simulink model "ame532Project1_Gimbal_Tracking_R2022aVersion"  (R2023a)
settings: Solver=ode4  StartTime=0.0  StopTime=60  FixedStep=0.01  RelTol=1e-3
model workspace (MAT data in the model file):
  theta : Simulink.Parameter (value not decoded)
values from neighbouring files (symbols this model uses):
  AR_s2 = b_s2/c_s2    [computeSurfacePos.m]
  AR_s3 = b_s3/c_s3    [computeSurfacePos.m]
  AR_s4 = b_s4/c_s4    [computeSurfacePos.m]
  AR_s5 = b_s5/c_s5    [computeSurfacePos.m]
  area_s2 = c_s2 * b_s2    [computeSurfacePos.m]
  area_s3 = c_s3 * b_s3    [computeSurfacePos.m]
  area_s4 = c_s4 * b_s4    [computeSurfacePos.m]
  area_s5 = c_s5 * b_s5    [computeSurfacePos.m]
  c_s2 = componentMassesAndGeom(3,2)    [computeSurfacePos.m]
  c_s3 = componentMassesAndGeom(4,2)    [computeSurfacePos.m]
  c_s4 = componentMassesAndGeom(1,2)    [computeSurfacePos.m]
  c_s5 = componentMassesAndGeom(2,2)    [computeSurfacePos.m]
undefined symbols (not defined in the file or in its folder): a0_s2, a0_s3, a0_s4, a0_s5, CD0_s2, CD0_s3, CD0_s4, CD0_s5, CDa_s2, CDa_s3, CDa_s4, CDa_s5, CL0_s2, CL0_s3, CL0_s4, CL0_s5, CM0_s2, CM0_s3, CM0_s4, CM0_s5, CMa_s2, CMa_s3, CMa_s4, CMa_s5, e_s2, e_s3, e_s4, e_s5, earthRadius, i_s2, i_s3, i_s4, i_s5, Jxx, Jxy, Jxz, Jyx, Jyy, Jyz, Jzx, Jzy, Jzz, LL, MM, n_s2, n_s3, n_s4, n_s5, NN, rEarth, ro, x_S2_B_B, x_S3_B_B, x_S4_B_B, x_S5_B_B
libraries: simulink_extras x34, matrix_library x19, aerolibutil x7, aerolibfltsims x4, vrlib x3, aerolibtransform2 x2, sharedutil x1, simulink x1
(part 4 of 4)

== matlab function ame532Project1_Gimbal_Tracking_R2022aVersion/IMU  Aircraft dynamic sim1/aeroforce coefficient block/calculatie alpha ==
  data: i0 input; alpha output; v_B input; n_vector input; wind_w input; v_B_BA output; C_BN input
function [alpha,v_B_BA] = fcn(i0,v_B,n_vector,wind_w,C_BN)

alpha = zeros(4,1);
% this function calculates alpha that the aero surface sees

v_B_BA = v_B - C_BN*wind_w;

for i = 1:4
    alpha(i) = i0(i) - asin(dot(v_B_BA,n_vector(:,i))/norm(v_B_BA));
end

== matlab function ame532Project1_Gimbal_Tracking_R2022aVersion/IMU  Aircraft dynamic sim1/aeroforce coefficient block/extract matrix function ==
  data: aero_surface_matrix input; AR_matrix output
function AR_matrix = Extract_AR(aero_surface_matrix)

AR_matrix = aero_surface_matrix(:,7);
end

== matlab function ame532Project1_Gimbal_Tracking_R2022aVersion/IMU  Aircraft dynamic sim1/aeroforce coefficient block/extract matrix function1 ==
  data: aero_surface_matrix input; AR_matrix output
function AR_matrix = Extract_AR(aero_surface_matrix)

AR_matrix = aero_surface_matrix(:,7);
end

== matlab function ame532Project1_Gimbal_Tracking_R2022aVersion/IMU  Aircraft dynamic sim1/mass & aero property calculation/CG calculation ==
  data: M_matrix input; cg_x output; cg_y output; cg_z output
function [cg_x, cg_y, cg_z] = CG_calc(M_matrix)

mass_col = M_matrix(:,1);
x_col = M_matrix(:,5);
y_col = M_matrix(:,6);
z_col = M_matrix(:,7);

cg_x = sum(mass_col.*x_col)/(sum(mass_col));
cg_y = sum(mass_col.*y_col)/(sum(mass_col));
cg_z = sum(mass_col.*z_col)/(sum(mass_col));

end

== matlab function ame532Project1_Gimbal_Tracking_R2022aVersion/IMU  Aircraft dynamic sim1/mass & aero property calculation/MATLAB Function ==
  data: cg_location input; M_matrix input; J_matrix output
function J_matrix = fcn(cg_location,M_matrix)


mass_col = M_matrix(:,1);
x_dim = M_matrix(:,2);
y_dim = M_matrix(:,3);
z_dim = M_matrix(:,4);
x_loc = M_matrix(:,5);
y_loc = M_matrix(:,6);
z_loc = M_matrix(:,7);

Ixx = zeros(11,1);
Iyy = zeros(11,1);
Izz = zeros(11,1);
Ixz = zeros(11,1);
Izx = Ixz;
Ixy = zeros(11,1);
Iyx = Ixy;
Iyz = zeros(11,1);
Izy = Iyz;

J_matrix = zeros(3,3);

% all moment of inertial is calculated wrt to CG

for i = 1:11
    Ixx(i) = mass_col(i)*(y_dim(i)^2+z_dim(i)^2)/(12)+mass_col(i)*((y_loc(i)-cg_location(2))^2+(z_loc(i)-cg_location(3))^2); % check discussion post
    Iyy(i) = mass_col(i)*(x_dim(i)^2+z_dim(i)^2)/(12)+mass_col(i)*((x_loc(i)-cg_location(1))^2+(z_loc(i)-cg_location(3))^2);
    Izz(i) = mass_col(i)*(y_dim(i)^2+x_dim(i)^2)/(12)+mass_col(i)*((y_loc(i)-cg_location(2))^2+(x_loc(i)-cg_location(1))^2);
    Ixz(i) = mass_col(i)*((z_loc(i)-cg_location(3))*(x_loc(i)-cg_location(1)));
    Ixy(i) = mass_col(i)*((x_loc(i)-cg_location(1))*(y_loc(i)-cg_location(2)));
    Iyz(i) = mass_col(i)*((y_loc(i)-cg_location(2))*(z_loc(i)-cg_location(3)));


end

J_matrix(1,1) = sum(Ixx);
J_matrix(2,2) = sum(Iyy);
J_matrix(3,3) = sum(Izz);
J_matrix(1,2) = sum(Ixy);
J_matrix(2,1) = sum(Ixy);
J_matrix(1,3) = sum(Ixz);
J_matrix(3,1) = sum(Ixz);
J_matrix(2,3) = sum(Iyz);
J_matrix(3,2) = sum(Iyz);

J_matrix = J_matrix./1000;
end

== matlab function ame532Project1_Gimbal_Tracking_R2022aVersion/IMU  Aircraft dynamic sim1/mass & aero property calculation/MATLAB Function1 ==
  data: aero_prop_matrix input; m_matrix input; x_b_s_ac output; cg_location input
function x_b_s_ac = calculate_x_b_sb(aero_prop_matrix,m_matrix,cg_location)
%this function calculates vector of each component to CM of aircraft

x_b_sb = zeros(3,4);
x_b_s_ac = zeros(3,4);
for i = 1:4
    x_b_s_ac(:,i) = m_matrix(i,5:7)' + [0.25*aero_prop_matrix(i,4) 0 0]';
    x_b_s_ac(:,i) = x_b_s_ac(:,i)- cg_location;

%     x_b_sb(:,i) = m_matrix(i,5:7)' - cg_location;

end

== matlab function ame532Project1_Gimbal_Tracking_R2022aVersion/Gimbal Aircraft dynamic sim/Rotational Kinematics/MATLAB Function2 ==
  data: phi input; H_matrix_inv output; theta input; psi input
function H_matrix_inv = inv_h_matrix_from_euler(phi,theta,psi)

H_matrix_inv = [1, tan(theta)*sin(phi), tan(theta)*cos(phi);
                0,      cos(phi),           -sin(phi);      
                0,     sin(phi)/cos(theta),   cos(phi)/cos(theta)];

end

== matlab function ame532Project1_Gimbal_Tracking_R2022aVersion/IMU  Aircraft dynamic sim1/mass & aero property calculation/MATLAB Function2 ==
  data: M_matrix input; aero_prop output
function aero_prop = fcn(M_matrix)

aero_prop = zeros(4,7);
for i = 1:4
    aero_prop(i,1:3) = M_matrix(i,5:7);
    aero_prop(i,4) = M_matrix(i,2);
end

%% define span for each surface

    aero_prop(1,5) = M_matrix(1,3); %right wing
    aero_prop(2,5) = M_matrix(2,3); %left wing
    aero_prop(3,5) = M_matrix(3,3); %hor stab.
    aero_prop(4,5) = M_matrix(4,4); %ver stab.
%% define area and aspect ratio for each surface

for i = 1:4
    aero_prop(i,6) = aero_prop(i,4)*aero_prop(i,5);
    aero_prop(i,7) = aero_prop(i,5)/aero_prop(i,4);
end

== matlab function ame532Project1_Gimbal_Tracking_R2022aVersion/IMU  Aircraft dynamic sim1/measurement subsystem/MATLAB Function ==
  data: velocity input; magnitude output
function magnitude = magnitude_from_vector(velocity)

magnitude = sqrt(velocity(1)^2+velocity(2)^2+velocity(3)^2);

end

== matlab function ame532Project1_Gimbal_Tracking_R2022aVersion/IMU  Aircraft dynamic sim1/translational dynamics/MATLAB Function10 ==
  data: p input; Cross_Product_Matrix output; q input; r input
function Cross_Product_Matrix = omega_to_cross_product_matrix(p,q,r)

    Cross_Product_Matrix =[0 -r q; r 0 -p; -q p 0];

end

== matlab function ame532Project1_Gimbal_Tracking_R2022aVersion/Gimbal system/magnitude ==
  data: x_E_BG input; R output
function R = fcn(x_E_BG)

R = sqrt(x_E_BG(1)^2+x_E_BG(2)^2+x_E_BG(3)^2);

== matlab function ame532Project1_Gimbal_Tracking_R2022aVersion/JeoIMUmodel/Aero Forces and Moments/F&M Horiz Stab Surface (S2)/Compute Aero Lift and Drag ==
  data: v_B_E_B input; alphaLocal output; v_B_A_B input; liftSurf output; dragSurf output; AR_s2 input; i_s2 input; n_s2 input; CL0_s2 input; CD0_s2 input; CDa_s2 input; a0_s2 input; e_s2 input; ro input; area_s2 input
function [alphaLocal, liftSurf, dragSurf] = fcn(v_B_E_B, v_B_A_B, AR_s2, i_s2, n_s2, CL0_s2, CD0_s2, CDa_s2, a0_s2, e_s2, ro, area_s2)
% Compute the lift and drag forces at the respective surface
% arSurf -> Aspect Ratio of respective surfaace
% ro -> air density (note: varies with altitude)
% v_infSurf -> total airspeed at the surface, i.e. Velocity of body w.r.t Inertial/ECEF as
% measured in body frame (|V_B_E_B|)
% v_B_A_B -> relative airspeed, where it is typically 
% v_B_E_B - c_B_N * v_A_N_N and v_A_N_N is the velocity of air mass w.r.t. NED 
% nSurf_B -> Normal force applied at surface
% eSurf -> Oswald efficiency
% alphaLocal0 -> Minimum drag Angle of Attack

v_infSurf = norm(v_B_E_B);
cSurfLocAlpha = 2*pi * (AR_s2/(2+AR_s2)); % Lift coefficient at the respective surface due to the local alpha (Angle of Attack)
alphaLocal = i_s2 - asin(dot(v_B_A_B,n_s2)/norm(v_B_A_B)); % in Radians
cSurfLift = CL0_s2 + cSurfLocAlpha * alphaLocal; % Lift coefficient of surface
cSurfDrag = CD0_s2 + CDa_s2 *(alphaLocal - a0_s2)^2 + (cSurfLift^2/(pi*e_s2*AR_s2));

liftSurf = cSurfLift * 0.5 * ro * (v_infSurf^2)*area_s2;
dragSurf = cSurfDrag * 0.5 * ro * (v_infSurf^2)*area_s2;

== matlab function ame532Project1_Gimbal_Tracking_R2022aVersion/JeoIMUmodel/Aero Forces and Moments/F&M Horiz Stab Surface (S2)/Compute Aero Moment ==
  data: v_B_E_B input; momSurf output; alphaLocal input; CM0_s2 input; CMa_s2 input; ro input; area_s2 input; c_s2 input
function momSurf = fcn(v_B_E_B, alphaLocal, CM0_s2, CMa_s2, ro, area_s2, c_s2)
% Compute the Moment at the respective Surface
% v_infSurf -> total airspeed at the surface, i.e. Velocity of body w.r.t Inertial/ECEF as
% measured in body frame (|V_B_E_B|)
% ro -> air density (note: varies with altitude)
% chordSurf -> Chord of the surface area
% cSurfM0 -> Initial moment coefficient of surface
% cSurfMalpha -> Moment coefficient at the respective surface due to the
% local alpha (Angle of Attack)
v_infSurf = norm(v_B_E_B);
cSurfMom = CM0_s2 + CMa_s2*alphaLocal; % Moment coefficient of surface
momSurf = cSurfMom * 0.5 * ro * (v_infSurf^2)*area_s2 * c_s2;

== matlab function ame532Project1_Gimbal_Tracking_R2022aVersion/JeoIMUmodel/Aero Forces and Moments/F&M Horiz Stab Surface (S2)/F&M in Body/Force Due to Lift and Drag ==
  data: lift input; forceLiftDragS2_B output; drag input; v_B_E_B input; n_s2 input
function forceLiftDragS2_B = fcn(lift, drag, v_B_E_B, n_s2)

forceLiftDrag_w = lift*n_s2 - [drag; 0; 0];
alpha = atan2(v_B_E_B(3), v_B_E_B(1));
beta = asin(v_B_E_B(2) / norm(v_B_E_B));

c_S_B = [cos(alpha), 0, sin(alpha); 0, 1, 0; -sin(alpha), 0, cos(alpha)] ;
c_W_S = [cos(beta), sin(beta), 0; -sin(beta), cos(beta), 0; 0,0,1];
c_W_B = c_W_S * c_S_B;

forceLiftDragS2_B = c_W_B' * forceLiftDrag_w;

== matlab function ame532Project1_Gimbal_Tracking_R2022aVersion/JeoIMUmodel/Aero Forces and Moments/F&M Horiz Stab Surface (S2)/F&M in Body/Moment S2 ==
  data: momSurf input; momS2_B output; FliftdragS input; n_s2 input; x_S2_B_B input
function momS2_B = fcn(momSurf, FliftdragS, n_s2, x_S2_B_B)
% Compute the moment at the respective surface
crot = [0,0,0; 0,0,-1; 0,1,0];

momS2_B = momSurf * crot* n_s2 + (cross(x_S2_B_B, FliftdragS));

== matlab function ame532Project1_Gimbal_Tracking_R2022aVersion/JeoIMUmodel/Aero Forces and Moments/F&M Horiz Stab Surface (S3)/Compute Aero Lift and Drag ==
  data: v_B_E_B input; alphaLocal output; v_B_A_B input; liftSurf output; dragSurf output; AR_s3 input; i_s3 input; n_s3 input; CL0_s3 input; CD0_s3 input; CDa_s3 input; a0_s3 input; e_s3 input; ro input; area_s3 input
function [alphaLocal, liftSurf, dragSurf] = fcn(v_B_E_B, v_B_A_B, AR_s3, i_s3, n_s3, CL0_s3, CD0_s3, CDa_s3, a0_s3, e_s3, ro, area_s3)
% Compute the lift and drag forces at the respective surface
% arSurf -> Aspect Ratio of respective surfaace
% ro -> air density (note: varies with altitude)
% v_infSurf -> total airspeed at the surface, i.e. Velocity of body w.r.t Inertial/ECEF as
% measured in body frame (|V_B_E_B|)
% v_B_A_B -> relative airspeed, where it is typically 
% v_B_E_B - c_B_N * v_A_N_N and v_A_N_N is the velocity of air mass w.r.t. NED 
% nSurf_B -> Normal force applied at surface
% eSurf -> Oswald efficiency
% alphaLocal0 -> Minimum drag Angle of Attack

v_infSurf = norm(v_B_E_B);
cSurfLocAlpha = 2*pi * (AR_s3/(2+AR_s3)); % Lift coefficient at the respective surface due to the local alpha (Angle of Attack)
alphaLocal = i_s3 - asin(dot(v_B_A_B,n_s3)/norm(v_B_A_B)); % in Radians
cSurfLift = CL0_s3 + cSurfLocAlpha * alphaLocal; % Lift coefficient of surface
cSurfDrag = CD0_s3 + CDa_s3 *(alphaLocal - a0_s3)^2 + (cSurfLift^2/(pi*e_s3*AR_s3));

liftSurf = cSurfLift * 0.5 * ro * (v_infSurf^2)*area_s3;
dragSurf = cSurfDrag * 0.5 * ro * (v_infSurf^2)*area_s3;

== matlab function ame532Project1_Gimbal_Tracking_R2022aVersion/Gimbal Aircraft dynamic sim/Rotational Kinematics/MATLAB Function3 ==
  data: p input; Cross_Product_Matrix output; q input; r input
function Cross_Product_Matrix = omega_to_cross_product_matrix(p,q,r)

    Cross_Product_Matrix =[0 -r q; r 0 -p; -q p 0];

end

== matlab function ame532Project1_Gimbal_Tracking_R2022aVersion/JeoIMUmodel/Aero Forces and Moments/F&M Horiz Stab Surface (S3)/Compute Aero Moment ==
  data: v_B_E_B input; momSurf output; alphaLocal input; CM0_s3 input; CMa_s3 input; ro input; area_s3 input; c_s3 input
function momSurf = fcn(v_B_E_B, alphaLocal, CM0_s3, CMa_s3, ro, area_s3, c_s3)
% Compute the Moment at the respective Surface
% v_infSurf -> total airspeed at the surface, i.e. Velocity of body w.r.t Inertial/ECEF as
% measured in body frame (|V_B_E_B|)
% ro -> air density (note: varies with altitude)
% chordSurf -> Chord of the surface area
% cSurfM0 -> Initial moment coefficient of surface
% cSurfMalpha -> Moment coefficient at the respective surface due to the
% local alpha (Angle of Attack)
v_infSurf = norm(v_B_E_B);
cSurfMom = CM0_s3 + CMa_s3*alphaLocal; % Moment coefficient of surface
momSurf = cSurfMom * 0.5 * ro * (v_infSurf^2)*area_s3 * c_s3;

== matlab function ame532Project1_Gimbal_Tracking_R2022aVersion/JeoIMUmodel/Aero Forces and Moments/F&M Horiz Stab Surface (S3)/F&M in Body/Force Due to Lift and Drag ==
  data: lift input; forceLiftDragS3_B output; drag input; v_B_E_B input; n_s3 input
function forceLiftDragS3_B = fcn(lift, drag, v_B_E_B, n_s3)

forceLiftDrag_w = lift*n_s3 - [drag; 0; 0];
alpha = atan2(v_B_E_B(3), v_B_E_B(1));
beta = asin(v_B_E_B(2) / norm(v_B_E_B));

c_S_B = [cos(alpha), 0, sin(alpha); 0, 1, 0; -sin(alpha), 0, cos(alpha)] ;
c_W_S = [cos(beta), sin(beta), 0; -sin(beta), cos(beta), 0; 0,0,1];
c_W_B = c_W_S * c_S_B;

forceLiftDragS3_B = c_W_B' * forceLiftDrag_w;

== matlab function ame532Project1_Gimbal_Tracking_R2022aVersion/JeoIMUmodel/Aero Forces and Moments/F&M Horiz Stab Surface (S3)/F&M in Body/Moment S3 ==
  data: momSurf input; momS3_B output; FliftdragS input; n_s3 input; x_S3_B_B input
function momS3_B = fcn(momSurf, FliftdragS, n_s3, x_S3_B_B)
% Compute the moment at the respective surface
crot = [0,0,0; 0,0,-1; 0,1,0];

momS3_B = momSurf * crot* n_s3 + (cross(x_S3_B_B, FliftdragS));

== matlab function ame532Project1_Gimbal_Tracking_R2022aVersion/JeoIMUmodel/Aero Forces and Moments/F&M Right Wing and Servo Surface (S4)/Compute Aero Lift and Drag ==
  data: v_B_E_B input; alphaLocal output; v_B_A_B input; liftSurf output; dragSurf output; AR_s4 input; i_s4 input; n_s4 input; CL0_s4 input; CD0_s4 input; CDa_s4 input; a0_s4 input; e_s4 input; ro input; area_s4 input
function [alphaLocal, liftSurf, dragSurf] = fcn(v_B_E_B, v_B_A_B, AR_s4, i_s4, n_s4, CL0_s4, CD0_s4, CDa_s4, a0_s4, e_s4, ro, area_s4)
% Compute the lift and drag forces at the respective surface
% arSurf -> Aspect Ratio of respective surfaace
% ro -> air density (note: varies with altitude)
% v_infSurf -> total airspeed at the surface, i.e. Velocity of body w.r.t Inertial/ECEF as
% measured in body frame (|V_B_E_B|)
% v_B_A_B -> relative airspeed, where it is typically 
% v_B_E_B - c_B_N * v_A_N_N and v_A_N_N is the velocity of air mass w.r.t. NED 
% nSurf_B -> Normal force applied at surface
% eSurf -> Oswald efficiency
% alphaLocal0 -> Minimum drag Angle of Attack

v_infSurf = norm(v_B_E_B);
cSurfLocAlpha = 2*pi * (AR_s4/(2+AR_s4)); % Lift coefficient at the respective surface due to the local alpha (Angle of Attack)
alphaLocal = i_s4 - asin(dot(v_B_A_B,n_s4)/norm(v_B_A_B)); % in Radians
cSurfLift = CL0_s4 + cSurfLocAlpha * alphaLocal; % Lift coefficient of surface
cSurfDrag = CD0_s4 + CDa_s4 *(alphaLocal - a0_s4)^2 + (cSurfLift^2/(pi*e_s4*AR_s4));

liftSurf = cSurfLift * 0.5 * ro * (v_infSurf^2)*area_s4;
dragSurf = cSurfDrag * 0.5 * ro * (v_infSurf^2)*area_s4;

== matlab function ame532Project1_Gimbal_Tracking_R2022aVersion/JeoIMUmodel/Aero Forces and Moments/F&M Right Wing and Servo Surface (S4)/Compute Aero Moment ==
  data: v_B_E_B input; momSurf output; alphaLocal input; CM0_s4 input; CMa_s4 input; ro input; area_s4 input; c_s4 input
function momSurf = fcn(v_B_E_B, alphaLocal, CM0_s4, CMa_s4, ro, area_s4, c_s4)
% Compute the Moment at the respective Surface
% v_infSurf -> total airspeed at the surface, i.e. Velocity of body w.r.t Inertial/ECEF as
% measured in body frame (|V_B_E_B|)
% ro -> air density (note: varies with altitude)
% chordSurf -> Chord of the surface area
% cSurfM0 -> Initial moment coefficient of surface
% cSurfMalpha -> Moment coefficient at the respective surface due to the
% local alpha (Angle of Attack)
v_infSurf = norm(v_B_E_B);
cSurfMom = CM0_s4 + CMa_s4*alphaLocal; % Moment coefficient of surface
momSurf = cSurfMom * 0.5 * ro * (v_infSurf^2)*area_s4 * c_s4;

== matlab function ame532Project1_Gimbal_Tracking_R2022aVersion/JeoIMUmodel/Aero Forces and Moments/F&M Right Wing and Servo Surface (S4)/F&M in Body/Force Due to Lift and Drag ==
  data: lift input; forceLiftDragS4_B output; drag input; v_B_E_B input; n_s4 input
function forceLiftDragS4_B = fcn(lift, drag, v_B_E_B, n_s4)

forceLiftDrag_w = lift*n_s4 - [drag; 0; 0];
alpha = atan2(v_B_E_B(3), v_B_E_B(1));
beta = asin(v_B_E_B(2) / norm(v_B_E_B));

c_S_B = [cos(alpha), 0, sin(alpha); 0, 1, 0; -sin(alpha), 0, cos(alpha)] ;
c_W_S = [cos(beta), sin(beta), 0; -sin(beta), cos(beta), 0; 0,0,1];
c_W_B = c_W_S * c_S_B;

forceLiftDragS4_B = c_W_B' * forceLiftDrag_w;

== matlab function ame532Project1_Gimbal_Tracking_R2022aVersion/Gimbal Aircraft dynamic sim/Rotational Kinematics/MATLAB Function4 ==
  data: DCM input; roll output; pitch output; yaw output
function [roll, pitch, yaw] = Euler_from_DCM(DCM)
   roll = atan2(DCM(2,3),DCM(3,3));
   pitch = -asin(DCM(1,3));
   yaw = atan2(DCM(1,2),DCM(1,1));
end

== matlab function ame532Project1_Gimbal_Tracking_R2022aVersion/JeoIMUmodel/Aero Forces and Moments/F&M Right Wing and Servo Surface (S4)/F&M in Body/Moment S4 ==
  data: momSurf input; momS4_B output; FliftdragS input; n_s4 input; x_S4_B_B input
function momS4_B = fcn(momSurf, FliftdragS, n_s4, x_S4_B_B)
% Compute the moment at the respective surface
crot = [0,0,0; 0,0,-1; 0,1,0];

momS4_B = momSurf * crot* n_s4 + (cross(x_S4_B_B, FliftdragS));

== matlab function ame532Project1_Gimbal_Tracking_R2022aVersion/JeoIMUmodel/Aero Forces and Moments/F&M Right Wing and Servo Surface (S5)/Compute Aero Lift and Drag ==
  data: v_B_E_B input; alphaLocal output; v_B_A_B input; liftSurf output; dragSurf output; AR_s5 input; i_s5 input; n_s5 input; CL0_s5 input; CD0_s5 input; CDa_s5 input; a0_s5 input; e_s5 input; ro input; area_s5 input
function [alphaLocal, liftSurf, dragSurf] = fcn(v_B_E_B, v_B_A_B, AR_s5, i_s5, n_s5, CL0_s5, CD0_s5, CDa_s5, a0_s5, e_s5, ro, area_s5)
% Compute the lift and drag forces at the respective surface
% arSurf -> Aspect Ratio of respective surfaace
% ro -> air density (note: varies with altitude)
% v_infSurf -> total airspeed at the surface, i.e. Velocity of body w.r.t Inertial/ECEF as
% measured in body frame (|V_B_E_B|)
% v_B_A_B -> relative airspeed, where it is typically 
% v_B_E_B - c_B_N * v_A_N_N and v_A_N_N is the velocity of air mass w.r.t. NED 
% nSurf_B -> Normal force applied at surface
% eSurf -> Oswald efficiency
% alphaLocal0 -> Minimum drag Angle of Attack

v_infSurf = norm(v_B_E_B);
cSurfLocAlpha = 2*pi * (AR_s5/(2+AR_s5)); % Lift coefficient at the respective surface due to the local alpha (Angle of Attack)
alphaLocal = i_s5 - asin(dot(v_B_A_B,n_s5)/norm(v_B_A_B)); % in Radians
cSurfLift = CL0_s5 + cSurfLocAlpha * alphaLocal; % Lift coefficient of surface
cSurfDrag = CD0_s5 + CDa_s5 *(alphaLocal - a0_s5)^2 + (cSurfLift^2/(pi*e_s5*AR_s5));

liftSurf = cSurfLift * 0.5 * ro * (v_infSurf^2)*area_s5;
dragSurf = cSurfDrag * 0.5 * ro * (v_infSurf^2)*area_s5;

== matlab function ame532Project1_Gimbal_Tracking_R2022aVersion/JeoIMUmodel/Aero Forces and Moments/F&M Right Wing and Servo Surface (S5)/Compute Aero Moment ==
  data: v_B_E_B input; momSurf output; alphaLocal input; CM0_s5 input; CMa_s5 input; ro input; area_s5 input; c_s5 input
function momSurf = fcn(v_B_E_B, alphaLocal, CM0_s5, CMa_s5, ro, area_s5, c_s5)
% Compute the Moment at the respective Surface
% v_infSurf -> total airspeed at the surface, i.e. Velocity of body w.r.t Inertial/ECEF as
% measured in body frame (|V_B_E_B|)
% ro -> air density (note: varies with altitude)
% chordSurf -> Chord of the surface area
% cSurfM0 -> Initial moment coefficient of surface
% cSurfMalpha -> Moment coefficient at the respective surface due to the
% local alpha (Angle of Attack)
v_infSurf = norm(v_B_E_B);
cSurfMom = CM0_s5 + CMa_s5*alphaLocal; % Moment coefficient of surface
momSurf = cSurfMom * 0.5 * ro * (v_infSurf^2)*area_s5 * c_s5;

== matlab function ame532Project1_Gimbal_Tracking_R2022aVersion/JeoIMUmodel/Aero Forces and Moments/F&M Right Wing and Servo Surface (S5)/F&M in Body/Force Due to Lift and Drag ==
  data: lift input; forceLiftDragS5_B output; drag input; v_B_E_B input; n_s5 input
function forceLiftDragS5_B = fcn(lift, drag, v_B_E_B, n_s5)

forceLiftDrag_w = lift*n_s5 - [drag; 0; 0];
alpha = atan2(v_B_E_B(3), v_B_E_B(1));
beta = asin(v_B_E_B(2) / norm(v_B_E_B));

c_S_B = [cos(alpha), 0, sin(alpha); 0, 1, 0; -sin(alpha), 0, cos(alpha)] ;
c_W_S = [cos(beta), sin(beta), 0; -sin(beta), cos(beta), 0; 0,0,1];
c_W_B = c_W_S * c_S_B;

forceLiftDragS5_B = c_W_B' * forceLiftDrag_w;

== matlab function ame532Project1_Gimbal_Tracking_R2022aVersion/JeoIMUmodel/Aero Forces and Moments/F&M Right Wing and Servo Surface (S5)/F&M in Body/Moment S5 ==
  data: momSurf input; momS5_B output; FliftdragS input; n_s5 input; x_S5_B_B input
function momS5_B = fcn(momSurf, FliftdragS, n_s5, x_S5_B_B)
% Compute the moment at the respective surface
crot = [0,0,0; 0,0,-1; 0,1,0];

momS5_B = momSurf * crot* n_s5 + (cross(x_S5_B_B, FliftdragS));

== matlab function ame532Project1_Gimbal_Tracking_R2022aVersion/JeoIMUmodel/Rotational Dynamics/Using Cross Product Matrix/Omega Cross Matrix ==
  data: PQR input; omegaMat output
function omegaMat = fcn(PQR)
P = PQR(1); % deg
Q = PQR(2); % deg
R = PQR(3); % deg
omegaMat = [0 -R Q; R 0 -P; -Q P 0];

== matlab function ame532Project1_Gimbal_Tracking_R2022aVersion/JeoIMUmodel/Rotational Kinematics_Quaternions/NormalizeQuaternion ==
  data: qin input; qoutNorm output
function qoutNorm = NormalizeQuaternion(qin)
qinMag = norm(qin);
qoutNorm = qin/qinMag;

== matlab function ame532Project1_Gimbal_Tracking_R2022aVersion/JeoIMUmodel/Rotational Kinematics_Quaternions/quaternionMultiplication ==
  data: q1 input; qResult output; q2 input
function qResult = quaternionMultiplication(q1,q2)
q1imag = [q1(2); q1(3); q1(4)] ;
q2imag = [q2(2); q2(3); q2(4)];
qResultMag = q1(1)*q2(1) - dot(q1imag, q2imag);

qResultVect = q1(1)*q2imag + q2(1)*q1imag + cross(q1imag,q2imag);
qResult = [qResultMag; qResultVect];
end

== matlab function ame532Project1_Gimbal_Tracking_R2022aVersion/JeoIMUmodel/Rotational Kinematics_Quaternions/quaternionToeuler ==
  data: qin input; yaw_deg output; pitch_deg output; roll_deg output
function [yaw_deg, pitch_deg, roll_deg] = quaternionsToEulerZYX(qin)
% Function to transfrom quaternion to Euler Angles in Tait-Bryan yaw,
% pitch, roll angle sequence

roll = atan2(2*(qin(1)*qin(2) + qin(3)*qin(4)), 1-2*(qin(2)^2 + qin(3)^2));
temp1 = sqrt(1+2*(qin(1)*qin(3)-qin(2)*qin(4)));
temp2 = sqrt(1-2*(qin(1)*qin(3) - qin(2)*qin(4)));
pitch = -pi/2 + 2*atan2(temp1, temp2);
yaw = atan2(2*(qin(1)*qin(4) + qin(2)*qin(3)) ,1-2*(qin(3)^2 + qin(4)^2));

yaw_deg = rad2deg(yaw);
pitch_deg = rad2deg(pitch);
roll_deg = rad2deg(roll);

end

== matlab function ame532Project1_Gimbal_Tracking_R2022aVersion/Gimbal Aircraft dynamic sim/Rotational Kinematics/C_EN1 ==
  data: roll input; ZYXDCM output; pitch input; yaw input
function ZYXDCM = DCM_from_Euler(roll,pitch,yaw) % sequence is yaw pitch roll
    yaw_matrix = [cos(yaw) sin(yaw) 0;
                  -sin(yaw) cos(yaw) 0;
                  0 0 1];
    pitch_matrix = [cos(pitch) 0 -sin(pitch);
                    0           1           0;
                    sin(pitch) 0  cos(pitch)];
    roll_matrix = [1            0           0;
                    0          cos(roll)    sin(roll);
                    0           -sin(roll)  cos(roll)];
    ZYXDCM = roll_matrix*pitch_matrix*yaw_matrix;
end

== matlab function ame532Project1_Gimbal_Tracking_R2022aVersion/JeoIMUmodel/Rotational Kinematics_Strapdown/Omega_B_N ==
  data: P_degPs input; y output; Q_degPs input; R_degPs input
function y = Omega_B_N(P_degPs,Q_degPs,R_degPs)
% Function used to generate cross product matrix of body rates (P,Q,R)
% w.r.t NED. This is basically a skew symmetric matrix
Omega_B_N = [0,-R_degPs,Q_degPs; R_degPs,0,-P_degPs; -Q_degPs,P_degPs,0];
y = Omega_B_N;

== matlab function ame532Project1_Gimbal_Tracking_R2022aVersion/JeoIMUmodel/Rotational Kinematics_Strapdown/dcmTOeuler ==
  data: inputDCM input; yaw_deg output; pitch_deg output; roll_deg output
function [yaw_deg, pitch_deg, roll_deg] = dcmTOEuler_TB(inputDCM)
% This function takes in a dcm and outputs the euler angles in a Tait-Bryan
% ZYX angle sequence
c12 = inputDCM(1,2);
c11 = inputDCM(1,1);
c13 = inputDCM(1,3);
c23 = inputDCM(2,3);
c33 = inputDCM(3,3);
yaw_deg = atand(c12/c11);
pitch_deg = -asind(c13);
roll_deg = atand(c23/c33);
end

== matlab function ame532Project1_Gimbal_Tracking_R2022aVersion/JeoIMUmodel/TransKin_RotKin_TansDynam/Rotational Kinematics_Euler/HinvMatrix ==
  data: pitchTheta input; hinv output; rollPhi input
function hinv = HinvMat(pitchTheta, rollPhi)
tThetasPhi = tan(pitchTheta) * sin(rollPhi);
tThetacPhi = tan(pitchTheta) * cos(rollPhi);
cPhi = cos(rollPhi);
sPhi = sin(rollPhi);
sPhiOvercTheta = sin(rollPhi)/cos(pitchTheta);
cPhiOvercTheta = cos(rollPhi)/cos(pitchTheta);

h = [1,tThetasPhi,tThetacPhi; 0,cPhi,-sPhi; 0,sPhiOvercTheta,cPhiOvercTheta];

hinv = h;

== matlab function ame532Project1_Gimbal_Tracking_R2022aVersion/JeoIMUmodel/TransKin_RotKin_TansDynam/Translational Kinematics/C_EN from LAX to ECEF ==
  data: lat input; ZYXDCM output; long input
function ZYXDCM = DCM_from_Euler(lat,long) % sequence of rotation is lat long
%     yaw_matrix = [cos(yaw) sin(yaw) 0;
%                   -sin(yaw) cos(yaw) 0;
%                   0 0 1];
    lat_matrix = [cos(lat) 0 -sin(lat);
                    0           1           0;
                    sin(lat) 0  cos(lat)];
    long_matrix = [1            0           0;
                    0          cos(-long)    sin(-long);
                    0           -sin(-long)  cos(-long)];

    adjust_matrix = [cos(pi/2) 0 -sin(pi/2);
                    0           1           0;
                    sin(pi/2) 0  cos(pi/2)];
    ZYXDCM = adjust_matrix*long_matrix*lat_matrix;
end

%this rotational matrix turns lat long coordinate into a new C_EN
%assuming the N CS is lat and longitudinally rotated, then you would do
%-longditudinal rotation then lat rotation, then rotate 90 degrees again to
%match ECEF

== matlab function ame532Project1_Gimbal_Tracking_R2022aVersion/JeoIMUmodel/TransKin_RotKin_TansDynam/Translational Kinematics/C_E_N ==
  data: lon_rad input; y output; lat_rad input
function y = NEDtoECEF(lon_rad, lat_rad)
% DCM to go from NED to ECEF frame

firstRot = [cos(lon_rad), cos(lon_rad), 0; -sin(lon_rad), cos(lon_rad), 0; 0, 0, 1;]; % Rotate about longitude first

secondRot = [0, 0, 1; 0, 1, 0; -1, 0,0]; % Left handed rotation of 90 deg 

thirdRot = [cos(lat_rad),0,sin(lat_rad); 0,1,0; -sin(lat_rad), 0, cos(lat_rad)];
% Multiply to get ECEF to NED DCM

c_NED_ECEF = thirdRot*secondRot*firstRot;
y = c_NED_ECEF';

== matlab function ame532Project1_Gimbal_Tracking_R2022aVersion/JeoIMUmodel/TransKin_RotKin_TansDynam/Translational Kinematics/c_B_N ==
  data: yaw_rad input; outDCM output; pitch_rad input; roll_rad input
function outDCM = euler2DCM_TB(yaw_rad, pitch_rad, roll_rad)
% This functions takes in yaw, pitch and roll angles to compute the
% Tait-Bryan ZYX sequence DCM from reference frame (NED) to Body Frame
yawDCM = [cos(yaw_rad), sin(yaw_rad), 0; -sin(yaw_rad), cos(yaw_rad), 0; 0, 0, 1];
pitchDCM = [cos(pitch_rad), 0, -sin(pitch_rad); 0, 1, 0; sin(pitch_rad), 0, cos(pitch_rad)];

rollDCM = [1,0,0; 0, cos(roll_rad), sin(roll_rad); 0, -sin(roll_rad), cos(roll_rad)];
%outDCM = yawDCM*pitchDCM*rollDCM;
outDCM = rollDCM*pitchDCM*yawDCM;
end

== matlab function ame532Project1_Gimbal_Tracking_R2022aVersion/Gimbal system/MATLAB Function2 ==
  data: phi input; H_matrix_inv output; theta input; psi input
function H_matrix_inv = inv_h_matrix_from_euler(phi,theta,psi)

H_matrix_inv = [1, tan(theta)*sin(phi), tan(theta)*cos(phi);
                0,      cos(phi),           -sin(phi);      
                0,     sin(phi)/cos(theta),   cos(phi)/cos(theta)];

end

== matlab function ame532Project1_Gimbal_Tracking_R2022aVersion/Gimbal system/Rotational Kinematics/C_BN ==
  data: roll input; ZYXDCM output; pitch input; yaw input
function ZYXDCM = DCM_from_Euler(roll,pitch,yaw) % sequence is yaw pitch roll
    yaw_matrix = [cos(yaw) sin(yaw) 0;
                  -sin(yaw) cos(yaw) 0;
                  0 0 1];
    pitch_matrix = [cos(pitch) 0 -sin(pitch);
                    0           1           0;
                    sin(pitch) 0  cos(pitch)];
    roll_matrix = [1            0           0;
                    0          cos(roll)    sin(roll);
                    0           -sin(roll)  cos(roll)];
    ZYXDCM = roll_matrix*pitch_matrix*yaw_matrix;
end

== matlab function ame532Project1_Gimbal_Tracking_R2022aVersion/Gimbal system/Rotational Kinematics/C_EN1 ==
  data: roll input; ZYXDCM output; pitch input; yaw input
function ZYXDCM = DCM_from_Euler(roll,pitch,yaw) % sequence is yaw pitch roll
    yaw_matrix = [cos(yaw) sin(yaw) 0;
                  -sin(yaw) cos(yaw) 0;
                  0 0 1];
    pitch_matrix = [cos(pitch) 0 -sin(pitch);
                    0           1           0;
                    sin(pitch) 0  cos(pitch)];
    roll_matrix = [1            0           0;
                    0          cos(roll)    sin(roll);
                    0           -sin(roll)  cos(roll)];
    ZYXDCM = roll_matrix*pitch_matrix*yaw_matrix;
end

== matlab function ame532Project1_Gimbal_Tracking_R2022aVersion/Gimbal system/Rotational Kinematics/C_EN2 ==
  data: roll input; ZYXDCM output; pitch input; yaw input
function ZYXDCM = DCM_from_Euler(roll,pitch,yaw) % sequence is yaw pitch roll
    yaw_matrix = [cos(yaw) -sin(yaw) 0;
                  sin(yaw) cos(yaw) 0;
                  0 0 1];
    pitch_matrix = [cos(pitch) 0 sin(pitch);
                    0           1           0;
                    -sin(pitch) 0  cos(pitch)];
    roll_matrix = [1            0           0;
                    0          cos(roll)    -sin(roll);
                    0           sin(roll)  cos(roll)];
    ZYXDCM = roll_matrix*pitch_matrix*yaw_matrix;
end
